simulink model "threeone"  (R2014b)
settings: Solver=ode45  StartTime=0.0  StopTime=10.0  RelTol=1e-3
settings Model: Creator=Administrator  LastModifiedBy=Administrator

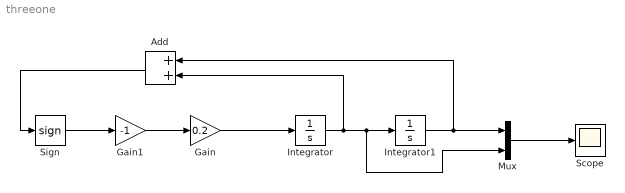
== system threeone ==
  Add : Sum
  Gain : Gain  Gain=0.2
  Gain1 : Gain  Gain=-1
  Integrator : Integrator  InitialCondition=1
  Integrator1 : Integrator
  Mux : Mux  Inputs=2
  Scope : Scope
  Sign : Signum
  wires:
  Integrator/1 -> Add/2, Mux/2, Integrator1/1
  Add/1 -> Sign/1
  Gain1/1 -> Gain/1
  Sign/1 -> Gain1/1
  Gain/1 -> Integrator/1
  Integrator1/1 -> Mux/1, Add/1
  Mux/1 -> Scope/1
